simulink model "disturbi_inner_sim"  (R2023b)
settings: Solver=VariableStepAuto  StartTime=0.0  StopTime=10.0  RelTol=1e-3
values from neighbouring files (symbols this model uses):
  A0 = [1 0 0; 0 0 1; 0 -1 0]*[0 0 1; 0 1 0; -1 0 0]    [planetary_phase_script.m]    (also in script_aocs.m = [0 0 1; 0 1 0; -1 0 0]; script_jupiter.m; simulation_inner1.m = A_b_n(:,:,end); srp_interplanetary.m = A_b_n(:,:,end))
  braccio_x = 2.7    [planetary_phase_script.m]    (also in script_aocs.m; script_jupiter.m; simulation_inner1.m; srp_interplanetary.m)
  braccio_y = 2.7    [planetary_phase_script.m]    (also in script_aocs.m; script_jupiter.m; simulation_inner1.m; srp_interplanetary.m)
  braccio_z = 3.2    [planetary_phase_script.m]    (also in script_aocs.m; script_jupiter.m; simulation_inner1.m; srp_interplanetary.m)
  gain_alphas = [-1000; -1000; -10]    [planetary_phase_script.m]    (also in script_aocs.m = [-100 -100 -1]'; script_jupiter.m; simulation_inner1.m = [-100 -100 -1]'; srp_interplanetary.m = [-100 -100 -1]')
  gain_integ = 0    [planetary_phase_script.m]    (also in script_aocs.m = -5; script_jupiter.m; simulation_inner1.m = -5; srp_interplanetary.m = -5)
  gain_omega = -1    [planetary_phase_script.m]    (also in script_aocs.m = -950; script_jupiter.m; simulation_inner1.m = -950; srp_interplanetary.m = -950)
  I = diag([11245.08 10044.71 17593.63])    [planetary_phase_script.m]    (also in script_aocs.m = [11245.08 0 0; 0 10044.71 0; 0 0 17593.63]; script_jupiter.m; simulation_inner1.m = [11245.08 0 0; 0 10044.71 0; 0 0 17593.63]; srp_interplanetary.m = [11245.08 0 0; 0 10044.71 0; 0 0 17593.63])
  I_inv = inv(I)    [planetary_phase_script.m]    (also in script_aocs.m; script_jupiter.m; simulation_inner1.m; srp_interplanetary.m)
  n = 2 * 2 * pi/60    (= 0.209439510239)    [planetary_phase_script.m]    (also in script_aocs.m = 0.10471975512; script_jupiter.m; simulation_inner1.m = 0.10471975512; srp_interplanetary.m = 0.10471975512)
  t_s = 1    [script_aocs.m]    (also in simulation_inner1.m; srp_interplanetary.m)
  T_srp_inner_x = Sr_medio/astroConstants(5) * A_cs/3 * ( 1 + q ) *  4.5    [srp_interplanetary.m]
  T_srp_inner_yy = Sr_medio/astroConstants(5) * A_cs/3 * ( 1 + q ) * 2 * delta_c_12    [srp_interplanetary.m]
  toll = deg2rad(15)    [planetary_phase_script.m]    (also in script_aocs.m; script_jupiter.m; simulation_inner1.m; srp_interplanetary.m)
  w0 = [0 0 n]    [planetary_phase_script.m]    (also in script_aocs.m; script_jupiter.m; simulation_inner1.m = w(:,end); srp_interplanetary.m = w(:,end))
libraries: simulink x3, matrix_library x1
(part 2 of 2)

== system disturbi_inner_sim/kinematics /kinematics 323/A323 matrix1/Subsystem2 ==
  angle : Inport
  Cos : Trigonometry  Operator=cos
  Sin : Trigonometry
  cos : Outport
  sin : Outport  Port=2
  wires:
  Cos/1 -> cos/1
  Sin/1 -> sin/1
  angle/1 -> Sin/1, Cos/1

== system disturbi_inner_sim/kinematics /kinematics 323/A323 matrix1/Subsystem3 ==
  angle : Inport
  Cos : Trigonometry  Operator=cos
  Sin : Trigonometry
  cos : Outport
  sin : Outport  Port=2
  wires:
  angle/1 -> Cos/1, Sin/1
  Sin/1 -> sin/1
  Cos/1 -> cos/1

== system disturbi_inner_sim/kinematics /logic 323/Subsystem4/If Action Subsystem ==
  In1 : Inport
  Action Port : ActionPort  ActionPortLabel=if(u1 == 1)
  Out1 : Outport
  wires:
  In1/1 -> Out1/1

== system disturbi_inner_sim/kinematics /logic 323/Subsystem4/If Action Subsystem1 ==
  In1 : Inport
  Action Port : ActionPort  ActionPortLabel=elseif(u1 == 0 & u3 == 0 & u4 == 1)
  Out1 : Outport
  wires:
  In1/1 -> Out1/1

== system disturbi_inner_sim/kinematics /logic 323/Subsystem4/If Action Subsystem2 ==
  In1 : Inport
  Action Port : ActionPort  ActionPortLabel=elseif( u1 == 0 & u2 == 0 & u3 == 1 & u4 == 0)
  Out1 : Outport
  wires:
  In1/1 -> Out1/1

== system disturbi_inner_sim/kinematics /logic 323/Subsystem4/If Action Subsystem3 ==
  In1 : Inport
  Action Port : ActionPort  ActionPortLabel=else
  Out1 : Outport
  wires:
  In1/1 -> Out1/1
